simulink model "10KW_PV_PSS_System"  (R2025a)
settings: Solver=VariableStepAuto  StartTime=0.0  StopTime=1.0  RelTol=1e-3
libraries: spsGroundLib x5, SignalEditorBlockLib x2, spsDCMachineLib x2, spsSeriesRLCBranchLib x2, spsVoltageMeasurementLib x2, spsCurrentMeasurementLib x1, spsDiodeLib x1, spsIGBTLib x1, sps_lib x1, spsPVArrayLib x1, eePwmGeneratorTwoLevel x1, spsThreePhaseSeriesRLCLoadLib x1
settings Model: Creator=shilp  LastModifiedBy=shilp
settings DebuggingCC: UnitsInconsistencyMsg=none

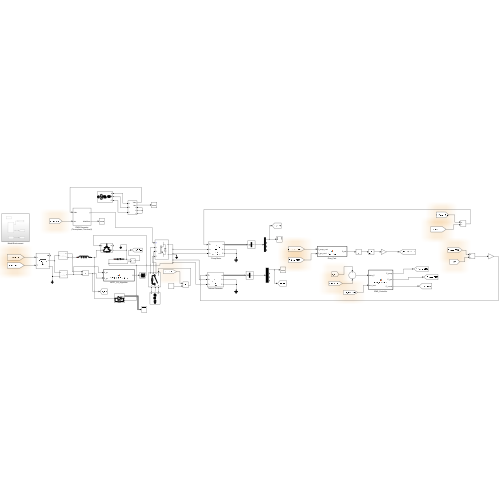
[thumbnail: Simulink's stored preview of the top-level diagram]
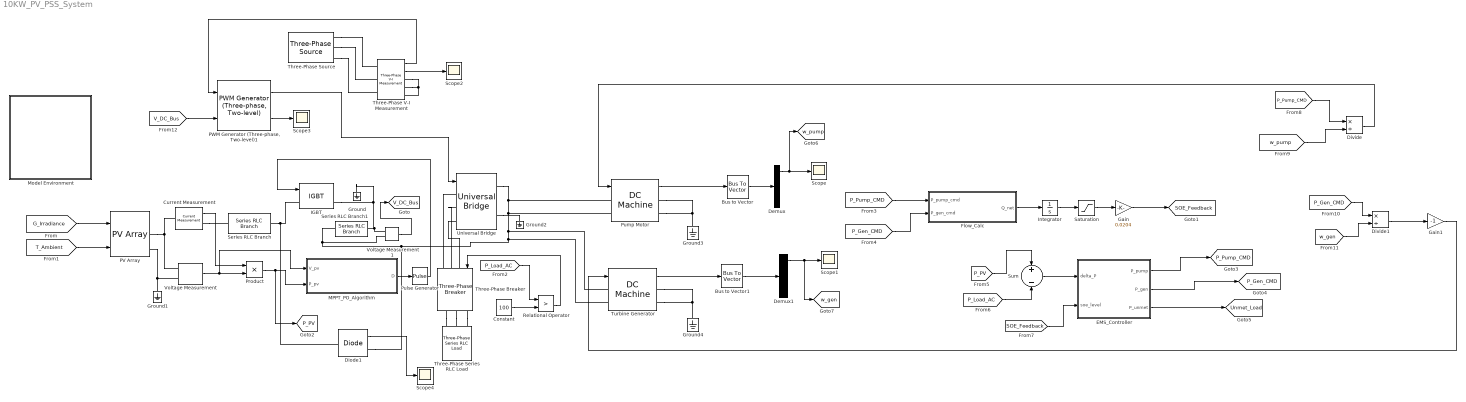
== system 10KW_PV_PSS_System ==
  Bus to Vector : BusToVector
  Bus to Vector1 : BusToVector
  Constant : Constant  Value=100
  Current Measurement : spsCurrentMeasurementLib/Current Measurement  PhasorSimulation=off  OutputType=Complex  PSBequivalent=0
  Demux : Demux
  Demux1 : Demux
  Diode1 : spsDiodeLib/Diode  Ron=0.001  Lon=0  Vf=0.8  IC=0  UseSnubber=0  Rs=500  Cs=250e-9  Measurements=on
  Divide : Product  Inputs=*/
  Divide1 : Product  Inputs=*/
  EMS_Controller : MATLAB Function  TreatAsAtomicUnit=on
  Flow_Calc : MATLAB Function  TreatAsAtomicUnit=on
  Gain : Gain  Gain=0.0204
  Gain1 : Gain  Gain=-1
  Ground{,1..4} (5 alike) : spsGroundLib/Ground  LConnTagsString=a
  IGBT : spsIGBTLib/IGBT  Ron=0.001  Lon=0  Vf=1  Tf=1e-6  Tt=2e-6  IC=0  Rs=1e5  Cs=inf  Measurements=on
  Integrator : Integrator  InitialCondition=2935
  MPPT_PO_Algorithm : MATLAB Function  TreatAsAtomicUnit=on
  Model Environment : Subsystem
  PV Array : spsPVArrayLib/PV Array  Npar=6  Nser=14  PlotType=array @ 1000 W/m2 & specified temperatures  S_vec="[ 1000  500  100 ]"  Temp_C_vec="[ 45 25  ]"  ModuleName=User-defined  PlotWhenSelected=off  Pm=213.15  Ncell=60  Voc=36.3  Isc=7.84  Vm=29  Im=7.35  beta_Voc_pc=-0.36099  alpha_Isc_pc=0.102  beta_Voc=-0.13104  alpha_Isc=0.0079968  IL=7.8654  I0=2.9273e-10  nI=0.98119  Rsh=313.0553  Rs=0.39381  RobustModel=off  RobustCellTemperature=313.3991  BAL=on  Tc=1e-6  Tfilter=5e-5
  "PWM Generator (Three-phase, Two-level)1" : eePwmGeneratorTwoLevel/PWM Generator (Three-phase, Two-level)  PWMMode=Continuous PWM (CPWM)  CPWMMode=SPWM: sinusoidal PWM  DPWMMode=60 DPWM: 60 degree discontinuous PWM  fsw=1e3  Ts=5e-5
      settings: LibrarySourceBlock=|
      | ee_sl_lib/Pulse Width
      | Modulation/PWM Generator
      | (Three-phase, Two-level)
  Product : Product
  Pulse Generator : DiscretePulseGenerator  PulseType=Time based  TimeSource=Use external signal  Period=0.0002  PulseWidth=25
  Pump Motor : spsDCMachineLib/DC Machine  PresetModel=No  MechanicalLoad=Torque TL  FieldType=Wound  ShowDetailedParameters=on  MeasurementBus=off  RLa="[ 0.6  0.012]"  RLf="[ 240  120]"  Laf=1.8  MachineConstant=Torque constant (N.m/A)  Ke=1.8  Kt=1.8  J=1  Bm=0  Tf=0  w0=1  Ifinit=0  TsPowergui=0  TsBlock=-1
  Relational Operator : RelationalOperator  Operator=>  OutDataTypeStr=boolean  RndMeth=Simplest  InputSameDT=off
  Saturation : Saturate  UpperLimit=5870  LowerLimit=0
  Scope{,1..4} (5 alike) : Scope
      Scope settings: ActiveDisplayYMinimum=0.9  ActiveDisplayYMaximum=1.1
      Scope1 settings: ActiveDisplayYMinimum=0.9  ActiveDisplayYMaximum=1.1
      Scope2 settings: ActiveDisplayYMinimum=-64.65650427548816  ActiveDisplayYMaximum=64.657200610170861  DataLoggingVariableName=ScopeData2
      Scope3 settings: ActiveDisplayYMinimum=-1.25  ActiveDisplayYMaximum=1.25  DataLoggingVariableName=ScopeData3
      Scope4 settings: ActiveDisplayYMinimum=-1  ActiveDisplayYMaximum=0.99999999999999989  DataLoggingVariableName=ScopeData4
  Series RLC Branch : spsSeriesRLCBranchLib/Series RLC Branch  LConnTagsString=__new0  RConnTagsString=__new0  BranchType=L  Resistance=1  Inductance=1e-3  SetiL0=off  InitialCurrent=0  Capacitance=1e-6  Setx0=off  InitialVoltage=0  Measurements=None
  Series RLC Branch1 : spsSeriesRLCBranchLib/Series RLC Branch  LConnTagsString=__new0  RConnTagsString=__new0  BranchType=C  Resistance=1  Inductance=1e-3  SetiL0=off  InitialCurrent=0  Capacitance=1e-6  Setx0=off  InitialVoltage=0  Measurements=None
  Sum : Sum  Inputs=+-
  Three-Phase Series RLC Load : spsThreePhaseSeriesRLCLoadLib/Three-Phase Series RLC Load  LConnTagsString=A|B|C  Configuration=Y (grounded)  NominalVoltage=1000  Vabc=[1e3 1e3 1e3]  Vabcp=[1e3 1e3 1e3]  NominalFrequency=60  UnbalancedPower=off  ActivePower=10e3  InductivePower=100  CapacitivePower=100  Pabc=[10e3 9e3 11e3]  QLabc=[100 90 110]  QCabc=[100 90 110]  Pabcp=[10e3 9e3 11e3]  QLabcp=[100 90 110]  QCabcp=[100 90 110]  Measurements=None  LoadType=constant Z
  Three-Phase V-I Measurement : spsThreePhaseVIMeasurementLib/Three-Phase V-I Measurement  VoltageMeasurement=phase-to-ground  SetLabelV=off  LabelV=Vabc  Vpu=off  VpuLL=off  CurrentMeasurement=yes  SetLabelI=off  LabelI=Iabc  Ipu=off  Pbase=100e6  Vbase=500e3  OutputType=Complex  PhasorSimulation=off  PSBequivalent=0
  Three-Phase Breaker : spsThreePhaseBreakerLib/Three-Phase Breaker  InitialState=open  SwitchA=on  SwitchB=on  SwitchC=on  SwitchTimes="[1/60  5/60]"  External=on  BreakerResistance=0.01  SnubberResistance=1e6  SnubberCapacitance=inf  Measurements=None
  Three-Phase Source : spsThreePhaseSourceLib/Three-Phase Source  InternalConnection=Yg  VoltagePhases=off  Voltage=400  PhaseAngle=0  Voltage_phases=[25e3 25e3 25e3]/sqrt(3)  PhaseAngles_phases=[0 -120 +120]  Frequency=60  NonIdealSource=on  SpecifyImpedance=off  Resistance=0.8929  Inductance=16.58e-3  ShortCircuitLevel=100e6  BaseVoltage=25e3  XRratio=7  BusType=swing  Pref=10e3  Qref=0  Prefabc=[10e3, 10e3, 10e3]  Qrefabc=[0, 0, 0]  Qmin=-inf  Qmax=inf
  Turbine Generator : spsDCMachineLib/DC Machine  PresetModel=No  MechanicalLoad=Torque TL  FieldType=Wound  ShowDetailedParameters=on  MeasurementBus=off  RLa="[ 0.6  0.012]"  RLf="[ 240  120]"  Laf=1.8  MachineConstant=Torque constant (N.m/A)  Ke=1.8  Kt=1.8  J=1  Bm=0  Tf=0  w0=1  Ifinit=0  TsPowergui=0  TsBlock=-1
  Universal Bridge : spsUniversalBridgeLib/Universal Bridge  Arms=3  SnubberResistance=1e5  SnubberCapacitance=inf  Device=IGBT / Diodes  Ron=1e-3  Lon=0  ForwardVoltages="[  0  0  ]"  ForwardVoltage=0  GTOparameters=[ 10e-6 , 20e-6 ]  IGBTparameters=[ 1e-6 , 2e-6 ]  Measurements=None  Measurements_2=None  converterType=Rectifier
  Voltage Measurement : spsVoltageMeasurementLib/Voltage Measurement  PhasorSimulation=off  OutputType=Complex  PSBequivalent=0
  Voltage Measurement1 : spsVoltageMeasurementLib/Voltage Measurement  PhasorSimulation=off  OutputType=Complex  PSBequivalent=0
  tag scope: P_Gen_CMD=global, P_PV=global, P_Pump_CMD=global, SOE_Feedback=global, Unmet_Load=global, V_DC_Bus=global, w_gen=global, w_pump=global
  wires:
  [G_Irradiance] -> PV Array/1
  [T_Ambient] -> PV Array/2
  Current Measurement/1 -> Product/1
  Voltage Measurement/1 -> MPPT_PO_Algorithm/1(V_pv), Product/2
  Product/1 -> [P_PV], MPPT_PO_Algorithm/2(P_pv)
  Pulse Generator/1 -> IGBT/1
  MPPT_PO_Algorithm/1(D) -> Pulse Generator/1
  [P_Load_AC] -> Relational Operator/1
  Relational Operator/1 -> Three-Phase Breaker/1
  Voltage Measurement1/1 -> [V_DC_Bus]
  Constant/1 -> Relational Operator/2
  Pump Motor/1 -> Bus to Vector/1
  Bus to Vector/1 -> Demux/1
  Turbine Generator/1 -> Bus to Vector1/1
  Bus to Vector1/1 -> Demux1/1
  Demux/1 -> Scope/1, [w_pump]
  Demux1/1 -> [w_gen], Scope1/1
  [P_Gen_CMD] -> Flow_Calc/2(P_gen_cmd)
  [P_Pump_CMD] -> Flow_Calc/1(P_pump_cmd)
  Flow_Calc/1(Q_net) -> Integrator/1
  Integrator/1 -> Saturation/1
  Saturation/1 -> Gain/1
  Gain/1 -> [SOE_Feedback]
  [P_PV] -> Sum/1
  [P_Load_AC] -> Sum/2
  EMS_Controller/1(P_pump) -> [P_Pump_CMD]
  EMS_Controller/2(P_gen) -> [P_Gen_CMD]
  EMS_Controller/3(P_unmet) -> [Unmet_Load]
  Sum/1 -> EMS_Controller/1(delta_P)
  [SOE_Feedback] -> EMS_Controller/2(soe_level)
  [P_Pump_CMD] -> Divide/1
  Divide/1 -> Pump Motor/1
  [P_Gen_CMD] -> Divide1/1
  [w_gen] -> Divide1/2
  Divide1/1 -> Gain1/1
  Gain1/1 -> Turbine Generator/1
  [w_pump] -> Divide/2
  Three-Phase V-I Measurement/1 -> "PWM Generator (Three-phase, Two-level)1"/1
  "PWM Generator (Three-phase, Two-level)1"/1 -> Universal Bridge/1
  Three-Phase V-I Measurement/2 -> Scope2/1
  [V_DC_Bus] -> "PWM Generator (Three-phase, Two-level)1"/2
  "PWM Generator (Three-phase, Two-level)1"/2 -> Scope3/1
  Diode1/1 -> Scope4/1
  connections:
  PV Array/RConn1 -- Voltage Measurement/LConn1 -- Current Measurement/LConn1
  PV Array/RConn2 -- Ground1/LConn1 -- Voltage Measurement/LConn2
  Current Measurement/RConn1 -- Series RLC Branch/LConn1
  Series RLC Branch/RConn1 -- IGBT/LConn1 -- Diode1/LConn1
  IGBT/RConn1 -- Voltage Measurement1/LConn1 -- Series RLC Branch1/RConn1 -- Ground/LConn1
  Universal Bridge/RConn2 -- Ground2/LConn1
  Three-Phase Breaker/RConn1 -- Three-Phase Series RLC Load/LConn3
  Three-Phase Breaker/RConn2 -- Three-Phase Series RLC Load/LConn2
  Three-Phase Breaker/RConn3 -- Three-Phase Series RLC Load/LConn1
  Universal Bridge/LConn1 -- Three-Phase Breaker/LConn3
  Universal Bridge/LConn2 -- Three-Phase Breaker/LConn2
  Universal Bridge/LConn3 -- Three-Phase Breaker/LConn1
  Voltage Measurement1/LConn2 -- Diode1/RConn1 -- Turbine Generator/LConn2 -- Turbine Generator/LConn1 -- Universal Bridge/RConn1 -- Pump Motor/LConn1 -- Pump Motor/LConn2 -- Series RLC Branch1/LConn1
  Pump Motor/RConn2 -- Ground3/LConn1 -- Pump Motor/RConn1
  Turbine Generator/RConn2 -- Ground4/LConn1 -- Turbine Generator/RConn1
  Three-Phase Source/RConn3 -- Three-Phase V-I Measurement/LConn3
  Three-Phase Source/RConn2 -- Three-Phase V-I Measurement/LConn2
  Three-Phase Source/RConn1 -- Three-Phase V-I Measurement/LConn1
  Three-Phase V-I Measurement/RConn1 -- Three-Phase V-I Measurement/RConn2 -- Three-Phase V-I Measurement/RConn3

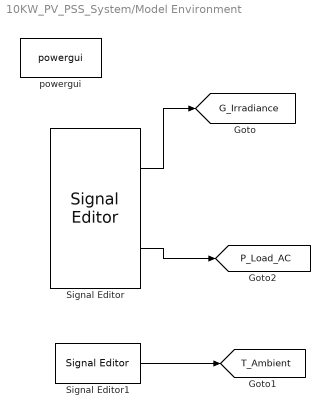
== system 10KW_PV_PSS_System/Model Environment ==
  Signal Editor : SignalEditorBlockLib/Signal Editor  FileName=C:\Users\shilp\Downloads\untitled.mat  ActiveScenario=Scenario  ActiveSignal=G_Irradiance  IsBus=off  OutputBusObjectStr=Bus: BusObject  SampleTime=86400  ZeroCross=off  OutputAfterFinalValue=Setting to zero  Unit=W/m^2  PreserveSignalName=on  ApplySigPropsToAllScenarios=off  ApplySigPropsToAllSignals=off  SignalPropertySource=Signal data in MAT file
  Signal Editor1 : SignalEditorBlockLib/Signal Editor  FileName=C:\Users\shilp\Downloads\untitleddd.mat  ActiveScenario=Scenario  ActiveSignal=T_Ambient  IsBus=off  OutputBusObjectStr=Bus: BusObject  SampleTime=0  ZeroCross=off  OutputAfterFinalValue=Setting to zero  Unit=inherit  PreserveSignalName=on  ApplySigPropsToAllScenarios=on  ApplySigPropsToAllSignals=off  SignalPropertySource=Dialog parameters
  powergui : sps_lib/powergui  Priority=1  SimulationMode=Discrete  SampleTime=5e-05  frequency=60  Iterations=50  frequencyindice=0  Pbase=100e6  ErrMax=1e-4  UnitsV=kV  UnitsW=MW  buscounter=0  FunctionMessages=off  echomessages=off  EnableUseOfTLC=off  CurrentSourceSwitches=off  DisableSnubberDevices=off  DisableRonSwitches=off  DisableVfSwitches=off  DisplayEquations=off  AutomaticDiscreteSolvers=off  SolverType=Tustin/Backward Euler (TBE)  Interpol=off  ExternalGateDelay=off  methode=off  Ts=100  x0status=blocks  SPID=on  SwTol=0  HookPort=off  NonlinearTolerance=1e-4  nMaxIteration=100  ContinueOnMaxIteration=off  RestoreLinks=warning  ResistiveCurrentMeasurement=off  Frange=[0:2:500]  Ylog=off  Xlog=on  ShowGrid=off  save=off  variable=ZData  structure=0  ZoomFFT=off  StartTime=0.0  cycles=1  DisplayStyle=1  fundamental=60  FreqAxis=off  MaxFrequency=1000  frequencyindicesteady=1  RmsSteady=1  display=off
  tag scope: G_Irradiance=global, P_Load_AC=global, T_Ambient=global
  wires:
  Signal Editor/1 -> [G_Irradiance]
  Signal Editor/2 -> [P_Load_AC]
  Signal Editor1/1 -> [T_Ambient]

== matlab function 10KW_PV_PSS_System/Flow_Calc ==
  data: P_pump_cmd input; P_gen_cmd input; Q_net output
function Q_net = Flow_Calc(P_pump_cmd, P_gen_cmd)

% Inputs:
% P_pump_cmd: Electrical power commanded by EMS for pumping (W)
% P_gen_cmd: Electrical power commanded by EMS for generating (W)

% Output:
% Q_net: Net flow rate change (m^3/s)

% --- PHYSICAL CONSTANTS (Based on a typical small PSS) ---
rho = 1000;      % Density of water (kg/m^3)
g = 9.81;        % Acceleration due to gravity (m/s^2)
H = 15;          % Assumed Net Hydraulic Head (Head must be substantial, e.g., 15 meters)
eta_pump = 0.70; % Pump/Motor efficiency (70%)
eta_turb = 0.75; % Turbine/Generator efficiency (75%)

% --- CALCULATE PUMP FLOW (Charging Mode) ---
% Formula: Q = P / (eta * rho * g * H)
if P_pump_cmd > 0
    Q_pump = P_pump_cmd / (eta_pump * rho * g * H);
else
    Q_pump = 0;
end

% --- CALCULATE GENERATOR FLOW (Discharging Mode) ---
% Note: Generating consumes water, so this flow is negative for the reservoir.
if P_gen_cmd > 0 
    Q_gen_needed = P_gen_cmd / (eta_turb * rho * g * H);
    % We use a negative sign because it removes water from the reservoir
    Q_gen = -Q_gen_needed;
else
    Q_gen = 0;
end

% --- CALCULATE NET FLOW RATE ---
% If pumping and generating happen at the same time, they cancel out flow.
Q_net = Q_pump + Q_gen;

end

== matlab function 10KW_PV_PSS_System/MPPT_PO_Algorithm ==
  data: V_pv input; D output; P_pv input
function D = MPPT_PO_Algorithm(V_pv, P_pv)

% Inputs:
% V_pv: Voltage of the PV Array (V)
% P_pv: Power of the PV Array (W)

% Output:
% D: Duty Cycle (0 to 1)

% --- PERSISTENT VARIABLES (Needed to remember past values) ---
% These variables retain their values between simulation steps.
persistent V_old P_old D_old;

% --- P&O Parameters ---
% Step size for perturbation (how much to change D each time)
D_step = 0.0005; 

% Initialization: Set initial values on the first step
if isempty(V_old)
    V_old = 0; 
    P_old = 0; 
    D_old = 0.5; % Start with a 50% duty cycle
end

% --- P&O LOGIC CORE ---

% 1. OBSERVE changes in Power (dP) and Voltage (dV)
dV = V_pv - V_old;
dP = P_pv - P_old;

% 2. DECIDE: Check the change in power to adjust the duty cycle (D)

if dP > 0 % Power is INCREASING
    
    if dV > 0 % V is increasing (Operating point moved in the RIGHT direction)
        D = D_old - D_step; % Decrease D to increase V (Boost Converter specific)
    else % V is decreasing (Operating point moved in the WRONG direction)
        D = D_old + D_step; % Increase D to decrease V
    end
    
elseif dP < 0 % Power is DECREASING
    
    if dV > 0 % V is increasing (Operating point moved in the WRONG direction)
        D = D_old + D_step; % Increase D to decrease V
    else % V is decreasing (Operating point moved in the RIGHT direction)
        D = D_old - D_step; % Decrease D to increase V
    end
    
else % dP == 0 (We are already at or near the MPPT)
    D = D_old;
    
end

% --- 3. APPLY CONSTRAINTS ---
% Ensure the duty cycle stays within physical limits (0.1 to 0.9 is safer than 0 to 1)
if D > 0.95
    D = 0.95; 
elseif D < 0.05
    D = 0.05;
end

% --- 4. UPDATE for next step ---
V_old = V_pv;
P_old = P_pv;
D_old = D;

end

== matlab function 10KW_PV_PSS_System/EMS_Controller ==
  data: delta_P input; P_pump output; soe_level input; P_gen output; P_unmet output
function [P_pump, P_gen, P_unmet] = EMS_Controller(delta_P, soe_level)

% Inputs:
% delta_P: Power Imbalance (P_pv - P_load)
% soe_level: Current State of Energy (kWh)

% Outputs:
% P_pump: Power command to the pump (W)
% P_gen: Power command to the generator (W)
% P_unmet: Unmet load (W)

% --- 1. DEFINE CONSTANTS ---
% Total storage capacity (from V_max calculation)
SOE_MAX = 120000;  % Example: 120 kWh in Watts-hours
SOE_MIN = 10000;   % Example: 10 kWh (minimum reserve)
TOL = 100;         % Tolerance (W) to prevent rapid switching

% --- 2. INITIALIZE OUTPUTS (Default: IDLE State) ---
P_pump = 0;
P_gen = 0;
P_unmet = 0;

% --- 3. APPLY LOGIC ---

% A. SYSTEM SURPLUS (delta_P > 0) -> PUMPING DECISION
if delta_P > TOL 
    
    if soe_level < SOE_MAX 
        % If not full, PUMP the entire surplus power
        P_pump = delta_P;
        
    else
        % If full, excess power is curtailed (or lost)
        % P_pump and P_gen remain 0
    end

% B. SYSTEM DEFICIT (delta_P < 0) -> GENERATING DECISION
elseif delta_P < -TOL
    
    required_power = abs(delta_P); % The power we need from storage
    
    if soe_level > SOE_MIN
        % If not empty, GENERATE the required power
        P_gen = required_power;
        
    else
        % If empty, we have UNMET LOAD
        P_unmet = required_power;
        % P_pump and P_gen remain 0
    end

% C. IDLE STATE (Near zero imbalance)
else
    % P_pump, P_gen, and P_unmet remain 0
end

end
